simulink library "lib_Wheels"  (R2017a)
settings: Solver=VariableStepAuto  StartTime=0.0  StopTime=10.0  RelTol=1e-3
undefined symbols (not defined in the file): Grade, time, Tire, Vehicle, whl
settings Model: Creator=Di Russo  LastModifiedBy=Vraj M

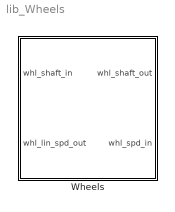
== system lib_Wheels ==
  Wheels : Subsystem
      mask Display:
      | image('Images/Wheel.jpg');
      | color('red');
      | port_label('input',1,'ShaftIn');
      | port_label('input',2,'SpdOut');
      | port_label('output',1,'ShaftOut');
      | port_label('output',2,'SpdIn');

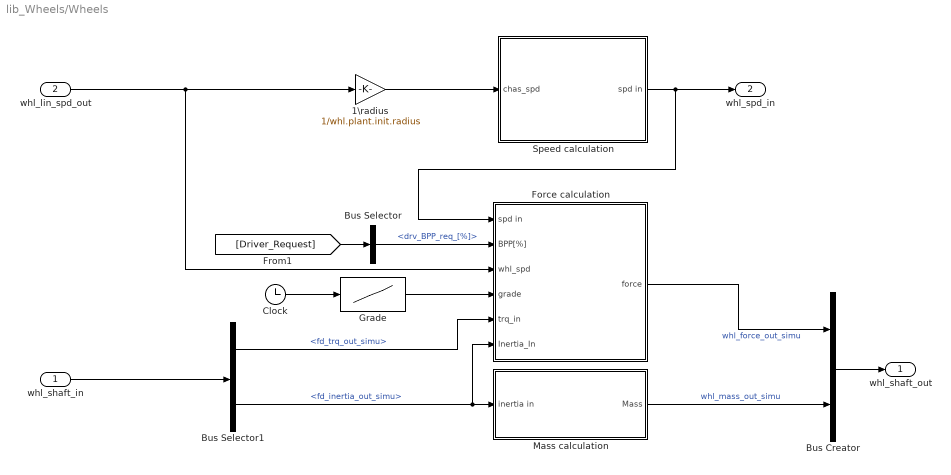
== system lib_Wheels/Wheels ==
  whl_shaft_in : Inport
  whl_lin_spd_out : Inport  Port=2
  "1\\radius " : Gain  Gain=1/whl.plant.init.radius  SaturateOnIntegerOverflow=on  OutDataTypeStr=Inherit: Same as input  ParamDataTypeStr=Inherit: Same as input
  Bus Creator : BusCreator  Inputs=2
  Bus Selector : BusSelector  OutputSignals=drv_BPP_req_[%]
  Bus Selector1 : BusSelector  OutputSignals=fd_trq_out_simu,fd_inertia_out_simu
  Clock : Clock
  Force calculation : Subsystem
  Grade : Lookup  InputValues=time  Table=Grade
  Mass calculation : Subsystem
  Speed calculation : Subsystem
  whl_shaft_out : Outport
  whl_spd_in : Outport  Port=2
  wires:
  Clock/1 -> Grade/1
  Grade/1 -> Force calculation/4(grade)
  Bus Creator/1 -> whl_shaft_out/1
  whl_shaft_in/1 -> Bus Selector1/1
  whl_lin_spd_out/1 -> "1\\radius "/1, Force calculation/3(whl_spd)
  Bus Selector1/2 -> Mass calculation/1(inertia in), Force calculation/6(Inertia_In)  "<fd_inertia_out_simu>"
  Bus Selector1/1 -> Force calculation/5(trq_in)  "<fd_trq_out_simu>"
  Mass calculation/1(Mass) -> Bus Creator/2  "whl_mass_out_simu"
  Speed calculation/1(spd in) -> whl_spd_in/1, Force calculation/1(spd in)
  Force calculation/1(force) -> Bus Creator/1  "whl_force_out_simu"
  "1\\radius "/1 -> Speed calculation/1(chas_spd)
  [Driver_Request] -> Bus Selector/1
  Bus Selector/1 -> Force calculation/2(BPP[%])  "<drv_BPP_req_[%]>"

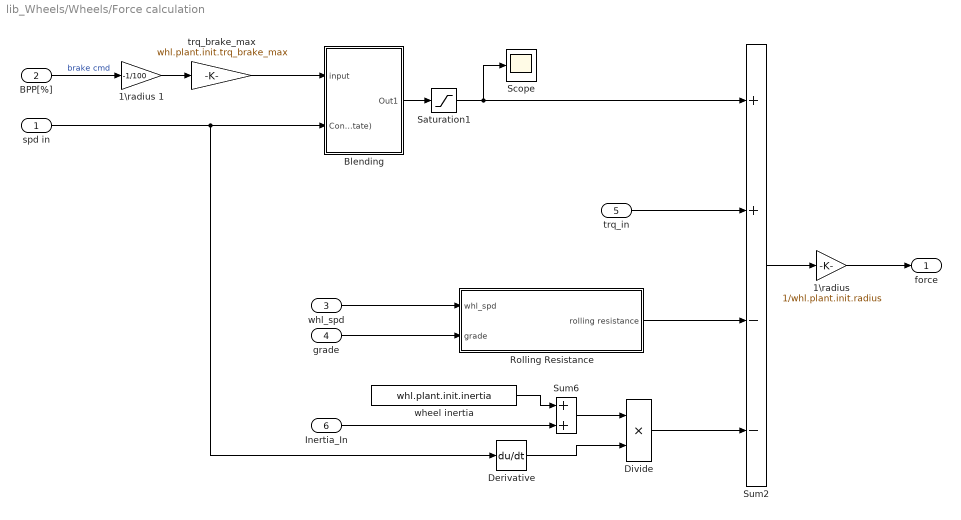
== system lib_Wheels/Wheels/Force calculation ==
  spd in : Inport
  BPP[%] : Inport  Port=2
  whl_spd : Inport  Port=3
  grade : Inport  Port=4
  trq_in : Inport  Port=5
  Inertia_In : Inport  Port=6
  "1\\radius " : Gain  Gain=1/whl.plant.init.radius  SaturateOnIntegerOverflow=on  OutDataTypeStr=Inherit: Same as input  ParamDataTypeStr=Inherit: Same as input
  1\radius 1 : Gain  Gain=-1/100  SaturateOnIntegerOverflow=on  OutDataTypeStr=Inherit: Same as input  ParamDataTypeStr=Inherit: Same as input
  Blending : Subsystem  mask(State dependent blending){xl=-0.1, yl=-1, xc=0, yc=0, xr=0.1, yr=1}
      mask prompts: xl "Left point (x-value):"; yl "Left point (y-value):"; xc "Center point (x-value):"; yc "Center point (y-value):"; xr "Right point (x-value):"; yr "Right point (y-vector):"
      mask Display: plot([-1 1 3 6 8], [1.5 1.5 0.5 4.0 4.0])
  Derivative : Derivative
  Divide : Product  Inputs=**
  Rolling Resistance : Subsystem
  Saturation1 : Saturate  UpperLimit=0  LowerLimit=-inf
  Scope : Scope
  Sum2 : Sum  Inputs=++--  SaturateOnIntegerOverflow=on  InputSameDT=on  OutDataTypeStr=Inherit: Same as first input
  Sum6 : Sum  SaturateOnIntegerOverflow=on  InputSameDT=on  OutDataTypeStr=Inherit: Same as first input
  trq_brake_max : Gain  Gain=whl.plant.init.trq_brake_max
  wheel inertia : Constant  Value=whl.plant.init.inertia
  force : Outport
  wires:
  Sum6/1 -> Divide/1
  wheel inertia/1 -> Sum6/1
  Divide/1 -> Sum2/4
  Derivative/1 -> Divide/2
  Inertia_In/1 -> Sum6/2
  Blending/1(Out1) -> Saturation1/1
  "1\\radius "/1 -> force/1
  1\radius 1/1 -> trq_brake_max/1
  trq_in/1 -> Sum2/2
  spd in/1 -> Blending/2(Control (state)), Derivative/1
  BPP[%]/1 -> 1\radius 1/1  "brake cmd"
  Saturation1/1 -> Sum2/1, Scope/1
  Sum2/1 -> "1\\radius "/1
  trq_brake_max/1 -> Blending/1(input)
  whl_spd/1 -> Rolling Resistance/1(whl_spd)
  grade/1 -> Rolling Resistance/2(grade)
  Rolling Resistance/1(rolling resistance) -> Sum2/3

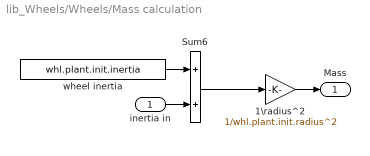
== system lib_Wheels/Wheels/Mass calculation ==
  inertia in : Inport
  1\radius^2 : Gain  Gain=1/whl.plant.init.radius^2  SaturateOnIntegerOverflow=on  OutDataTypeStr=Inherit: Same as input  ParamDataTypeStr=Inherit: Same as input
  Sum6 : Sum  SaturateOnIntegerOverflow=on  InputSameDT=on  OutDataTypeStr=Inherit: Same as first input
  wheel inertia : Constant  Value=whl.plant.init.inertia
  Mass : Outport
  wires:
  wheel inertia/1 -> Sum6/1
  Sum6/1 -> 1\radius^2/1
  1\radius^2/1 -> Mass/1
  inertia in/1 -> Sum6/2

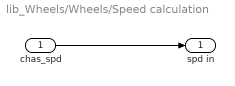
== system lib_Wheels/Wheels/Speed calculation ==
  chas_spd : Inport
  spd in : Outport
  wires:
  chas_spd/1 -> spd in/1

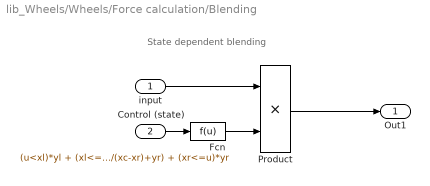
== system lib_Wheels/Wheels/Force calculation/Blending ==
  note: State dependent blending
  input : Inport
  Control (state) : Inport  Port=2
  Fcn : Fcn  Expr=(u<xl)*yl + (xl<=u)*(u<xc)*((yc-yl)*(u-xl)/(xc-xl)+yl) + (xc<=u)*(u<xr)*((yc-yr)*(u-xr)/(xc-xr)+yr) + (xr<=u)*yr
  Product : Product  SaturateOnIntegerOverflow=on  InputSameDT=on  OutDataTypeStr=Inherit: Same as first input
  Out1 : Outport
  wires:
  Fcn/1 -> Product/2
  Product/1 -> Out1/1
  Control (state)/1 -> Fcn/1
  input/1 -> Product/1

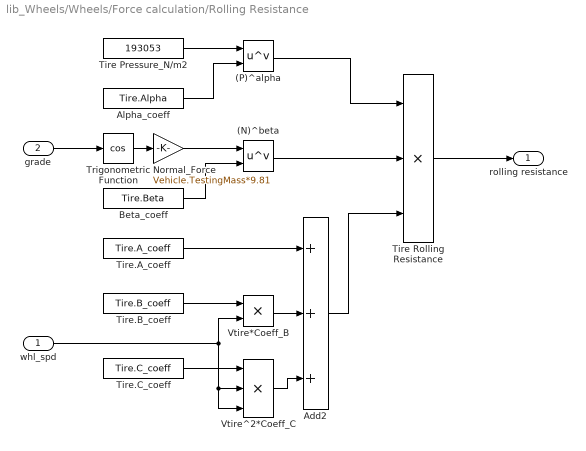
== system lib_Wheels/Wheels/Force calculation/Rolling Resistance ==
  whl_spd : Inport
  grade : Inport  Port=2
  (N)^beta : Math  Operator=pow  SaturateOnIntegerOverflow=on
  (P)^alpha : Math  Operator=pow  SaturateOnIntegerOverflow=on
  Add2 : Sum  Inputs=+++
  Alpha_coeff : Constant  Value=Tire.Alpha
  Beta_coeff : Constant  Value=Tire.Beta
  Normal_Force : Gain  Gain=Vehicle.TestingMass*9.81
  Tire Pressure_N/m2 : Constant  Value=193053
  Tire Rolling Resistance : Product  Inputs=***
  Tire.A_coeff : Constant  Value=Tire.A_coeff
  Tire.B_coeff : Constant  Value=Tire.B_coeff
  Tire.C_coeff : Constant  Value=Tire.C_coeff
  Trigonometric Function : Trigonometry  Operator=cos
  Vtire*Coeff_B : Product  Inputs=**
  Vtire^2*Coeff_C : Product  Inputs=***
  rolling resistance : Outport
  wires:
  Trigonometric Function/1 -> Normal_Force/1
  Tire Rolling Resistance/1 -> rolling resistance/1
  Add2/1 -> Tire Rolling Resistance/3
  Vtire*Coeff_B/1 -> Add2/2
  Vtire^2*Coeff_C/1 -> Add2/3
  Tire.C_coeff/1 -> Vtire^2*Coeff_C/1
  Tire.B_coeff/1 -> Vtire*Coeff_B/1
  Tire.A_coeff/1 -> Add2/1
  (N)^beta/1 -> Tire Rolling Resistance/2
  Beta_coeff/1 -> (N)^beta/2
  Normal_Force/1 -> (N)^beta/1
  (P)^alpha/1 -> Tire Rolling Resistance/1
  Alpha_coeff/1 -> (P)^alpha/2
  Tire Pressure_N/m2/1 -> (P)^alpha/1
  grade/1 -> Trigonometric Function/1
  whl_spd/1 -> Vtire^2*Coeff_C/2, Vtire^2*Coeff_C/3, Vtire*Coeff_B/2
